simulink model "foc_current_loop_verify"  (R2024a)
settings: Solver=FixedStepDiscrete  StartTime=0.0  StopTime=0.05  FixedStep=5e-05  RelTol=1e-3
undefined symbols (not defined in the file or in its folder): DiscIntNeverNeededParam
settings Model: Creator=黄钟锐  LastModifiedBy=黄钟锐
settings SFSimCC: SimCustomHeaderCode="#include \"simulink_foc_entry.h\""
settings SFSimCC: SimUserSources=|
  | D:\Documents\motor_control\src\sim\foc_sim.c
  | D:\Documents\motor_control\src\control\current_controller.c
  | D:\Documents\motor_control\src\control\velocity_controller.c
  | D:\Documents\motor_control\src\foc\foc_math.c
  | D:\Documents\motor_control\src\foc\svpwm.c
settings SFSimCC: SimUserIncludeDirs=|
  | D:\Documents\motor_control
  | D:\Documents\motor_control\include
  | D:\Documents\motor_control\src
  | D:\Documents\motor_control\src\foc
  | D:\Documents\motor_control\src\control
  | D:\Documents\motor_control\src\sim

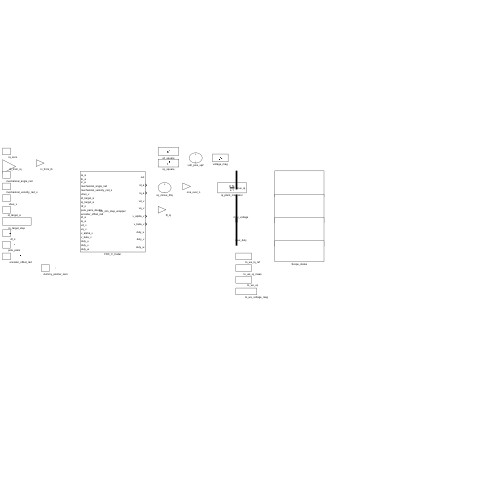
[thumbnail: Simulink's stored preview of the top-level diagram]
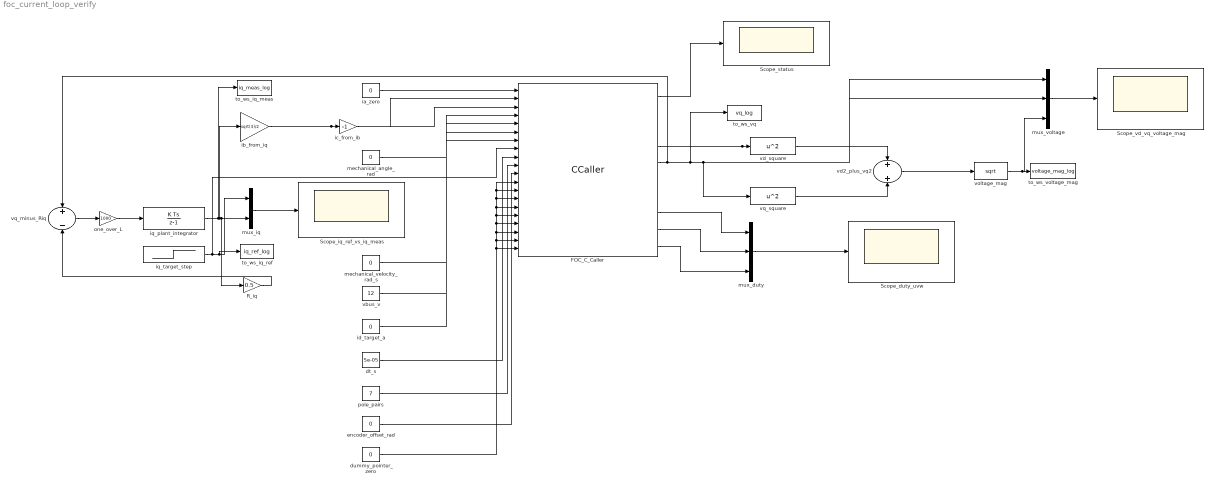
== system foc_current_loop_verify ==
  FOC_C_Caller : CCaller  FunctionName=foc_sim_step_wrapper  PortSpecificationStruct="%)30     .    8\"0   8    (     @         %    \"    !4    !     0         %  0 \"0    $    _    07)G3F%M90  4&]R=$YA;64 4V-O<&4     26YD97@     5'EP90      4VEZ90      27-';&]B86P   X    P    !@    @    $          4    (     0    ,    !         !   P!O=70 #@   #     &    \"     0         !0    @    !     P    $         $  # &]U=  .    .     8    (    !          %    \"     $    &     0         0  ...(+12198 chars)"
  R_iq : Gain  Gain=0.5
  Scope_duty_uvw : Scope
  Scope_iq_ref_vs_iq_meas : Scope
  Scope_status : Scope
  Scope_vd_vq_voltage_mag : Scope
  dt_s : Constant  Value=5e-05
  dummy_pointer_zero : Constant  Value=0
  encoder_offset_rad : Constant  Value=0
  ia_zero : Constant  Value=0
  ib_from_iq : Gain  Gain=sqrt(3)/2
  ic_from_ib : Gain  Gain=-1
  id_target_a : Constant  Value=0
  iq_plant_integrator : DiscreteIntegrator  gainval=1  SampleTime=5e-05  ICPrevOutput=DiscIntNeverNeededParam  ICPrevScaledInput=DiscIntNeverNeededParam
  iq_target_step : Step  Time=0.01  After=0.5  SampleTime=5e-05
  mechanical_angle_rad : Constant  Value=0
  mechanical_velocity_rad_s : Constant  Value=0
  mux_duty : Mux  Inputs=3
  mux_iq : Mux  Inputs=2
  mux_voltage : Mux  Inputs=3
  one_over_L : Gain  Gain=1000
  pole_pairs : Constant  Value=7
  to_ws_iq_meas : ToWorkspace  VariableName=iq_meas_log  SaveFormat=Timeseries  SampleTime=-1
  to_ws_iq_ref : ToWorkspace  VariableName=iq_ref_log  SaveFormat=Timeseries  SampleTime=-1
  to_ws_voltage_mag : ToWorkspace  VariableName=voltage_mag_log  SaveFormat=Timeseries  SampleTime=-1
  to_ws_vq : ToWorkspace  VariableName=vq_log  SaveFormat=Timeseries  SampleTime=-1
  vbus_v : Constant  Value=12
  vd2_plus_vq2 : Sum
  vd_square : Math  Operator=square
  voltage_mag : Sqrt
  vq_minus_Riq : Sum  Inputs=+-
  vq_square : Math  Operator=square
  wires:
  one_over_L/1 -> iq_plant_integrator/1
  vq_minus_Riq/1 -> one_over_L/1
  ia_zero/1 -> FOC_C_Caller/1
  iq_plant_integrator/1 -> R_iq/1, mux_iq/2, ib_from_iq/1, to_ws_iq_meas/1
  mux_iq/1 -> Scope_iq_ref_vs_iq_meas/1
  pole_pairs/1 -> FOC_C_Caller/10
  iq_target_step/1 -> mux_iq/1, to_ws_iq_ref/1, FOC_C_Caller/8
  ib_from_iq/1 -> FOC_C_Caller/2, ic_from_ib/1
  R_iq/1 -> vq_minus_Riq/2
  id_target_a/1 -> FOC_C_Caller/7
  mechanical_velocity_rad_s/1 -> FOC_C_Caller/5
  ic_from_ib/1 -> FOC_C_Caller/3
  vbus_v/1 -> FOC_C_Caller/6
  mechanical_angle_rad/1 -> FOC_C_Caller/4
  encoder_offset_rad/1 -> FOC_C_Caller/11
  dt_s/1 -> FOC_C_Caller/9
  dummy_pointer_zero/1 -> FOC_C_Caller/12, FOC_C_Caller/13, FOC_C_Caller/14, FOC_C_Caller/15, FOC_C_Caller/16, FOC_C_Caller/17, FOC_C_Caller/18, FOC_C_Caller/19, FOC_C_Caller/20
  FOC_C_Caller/9 -> mux_duty/2
  FOC_C_Caller/5 -> vq_square/1, mux_voltage/2, to_ws_vq/1, vq_minus_Riq/1
  FOC_C_Caller/1 -> Scope_status/1
  FOC_C_Caller/8 -> mux_duty/1
  FOC_C_Caller/4 -> mux_voltage/1, vd_square/1
  FOC_C_Caller/10 -> mux_duty/3
  vd_square/1 -> vd2_plus_vq2/1
  vd2_plus_vq2/1 -> voltage_mag/1
  vq_square/1 -> vd2_plus_vq2/2
  mux_duty/1 -> Scope_duty_uvw/1
  voltage_mag/1 -> mux_voltage/3, to_ws_voltage_mag/1
  mux_voltage/1 -> Scope_vd_vq_voltage_mag/1
